simulink model "accel"  (R2020b)
settings: Solver=VariableStepAuto  StartTime=0.0  StopTime=10.0  RelTol=1e-3
model mask{a_sf_cc=[1, 0, 0; 0, 1, 0; 0, 0, 1], a_bias=[0 0 0], a_noise=[0 0 0], a_sath=[inf inf inf], a_satl=[-inf -inf -inf], sample_rate=100}
  mask prompts: a_sf_cc "Scale Factors and cross coupling:"; a_bias "Bias [m/s/s]:"; a_noise "Noise [m/s/s]:"; a_sath "Upper limits [m/s/s]:"; a_satl "Lower limits [m/s/s]:"; sample_rate "Sample Rate [Hz]:"
model workspace (MAT data in the model file):
  a_bias = Simulink.Parameter
  a_bias.Value = [0 0 0]
  a_bias.DataType = 'auto'
  a_bias.Dimensions = [1 3]
  a_noise = Simulink.Parameter
  a_noise.Value = [0 0 0]
  a_noise.DataType = 'auto'
  a_noise.Dimensions = [1 3]
  a_sath = Simulink.Parameter
  a_sath.Value = [Inf Inf Inf]
  a_sath.DataType = 'auto'
  a_sath.Dimensions = [1 3]
  a_satl = Simulink.Parameter
  a_satl.Value = [-Inf -Inf -Inf]
  a_satl.DataType = 'auto'
  a_satl.Dimensions = [1 3]
  a_sf_cc = Simulink.Parameter
  a_sf_cc.Value = [1  0  0; 0  1  0; 0  0  1]
  a_sf_cc.DataType = 'auto'
  a_sf_cc.Dimensions = [3 3]
  sample_rate = Simulink.Parameter
  sample_rate.Value = 100
  sample_rate.DataType = 'auto'
  sample_rate.Dimensions = [1 1]
libraries: simulink x1
settings Model: ParameterArgumentNames=a_bias,a_noise,a_sath,a_satl,a_sf_cc,sample_rate  OrderedModelArguments=off  Creator=brian  LastModifiedBy=brian

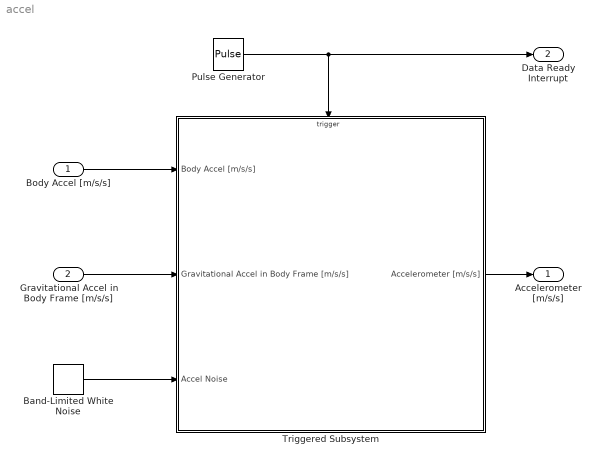
== system accel ==
  Body Accel [m/s/s] : Inport
  Gravitational Accel in Body Frame [m/s/s] : Inport  Port=2
  Band-Limited White Noise : simulink/Sources/Band-Limited White Noise  Cov=a_noise  Ts=0.1  seed=[23341]
  Pulse Generator : DiscretePulseGenerator  PulseType=Time based  Period=1/sample_rate  PulseWidth=5
  Triggered Subsystem : Subsystem  TreatAsAtomicUnit=on
  Accelerometer [m/s/s] : Outport
  Data Ready Interrupt : Outport  Port=2
  wires:
  Gravitational Accel in Body Frame [m/s/s]/1 -> Triggered Subsystem/2(Gravitational Accel in Body Frame [m/s/s])
  Pulse Generator/1 -> Data Ready Interrupt/1, Triggered Subsystem/Trigger
  Band-Limited White Noise/1 -> Triggered Subsystem/3(Accel Noise)
  Triggered Subsystem/1(Accelerometer [m/s/s]) -> Accelerometer [m/s/s]/1
  Body Accel [m/s/s]/1 -> Triggered Subsystem/1(Body Accel [m/s/s])

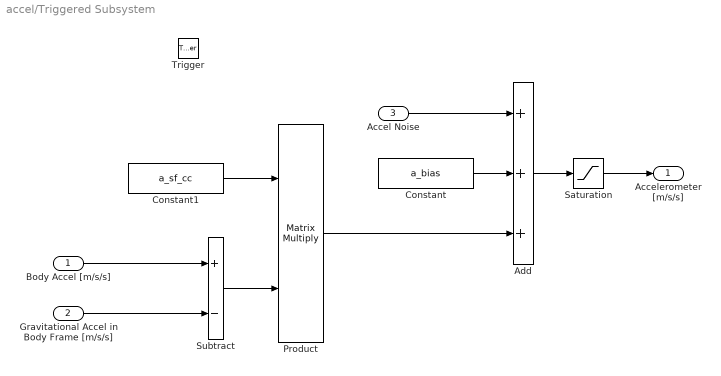
== system accel/Triggered Subsystem ==
  Body Accel [m/s/s] : Inport  PortDimensions=3
  Gravitational Accel in Body Frame [m/s/s] : Inport  Port=2  PortDimensions=3
  Accel Noise : Inport  Port=3  PortDimensions=3
  Trigger : TriggerPort  VariantControl=Variant
  Add : Sum  Inputs=+++
  Constant : Constant  Value=a_bias
  Constant1 : Constant  Value=a_sf_cc
  Product : Product  Multiplication=Matrix(*)
  Saturation : Saturate  UpperLimit=a_sath  LowerLimit=a_satl
  Subtract : Sum  Inputs=+-
  Accelerometer [m/s/s] : Outport  PortDimensions=3
  wires:
  Gravitational Accel in Body Frame [m/s/s]/1 -> Subtract/2
  Accel Noise/1 -> Add/1
  Constant/1 -> Add/2
  Product/1 -> Add/3
  Body Accel [m/s/s]/1 -> Subtract/1
  Add/1 -> Saturation/1
  Saturation/1 -> Accelerometer [m/s/s]/1
  Constant1/1 -> Product/1
  Subtract/1 -> Product/2
